simulink model "QAM"  (R2022b)
settings: Solver=VariableStepAuto  StartTime=0.0  StopTime=stop_time  RelTol=1e-3
libraries: commdigbbndam3 x2, commchan3 x1, commsink2 x1, commrandsrc3 x1
settings Model: Creator=g  LastModifiedBy=g

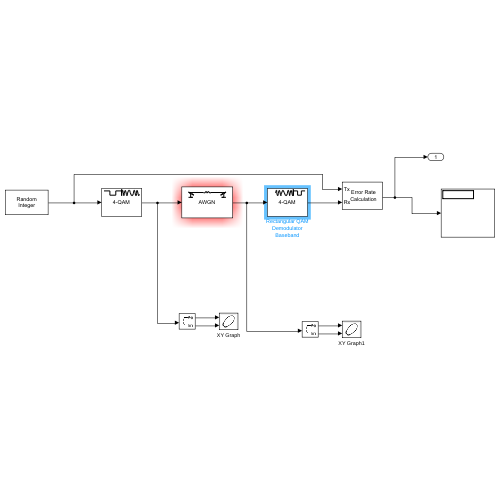
[thumbnail: Simulink's stored preview of the top-level diagram]
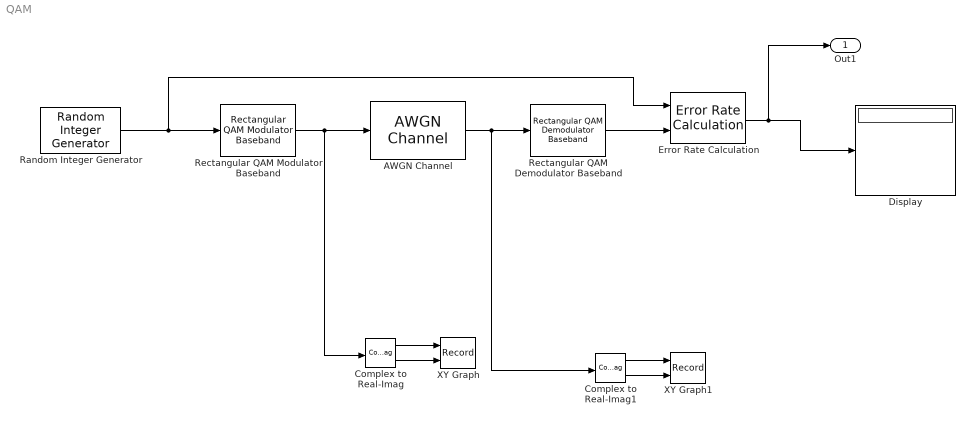
== system QAM ==
  AWGN Channel : commchan3/AWGN Channel  InputProcessing=Columns as channels (frame based)  seed=67  noiseMode="Signal to noise ratio  (Eb/No)"  EbNodB=Eb_No_db  EsNodB=10  SNRdB=10  bitsPerSym=2  Ps=1  Tsym=0.2  variance=1
  Complex to Real-Imag : ComplexToRealImag
  Complex to Real-Imag1 : ComplexToRealImag
  Display : Display
  Error Rate Calculation : commsink2/Error Rate Calculation  N=0  st_delay=0  cp_mode=Entire frame  subframe=[]  PMode=Port  WsName=ErrorVec  RsMode2=off  stop=off  numErr=100  maxBits=1e6
  Random Integer Generator : commrandsrc3/Random Integer Generator  SetSize=m_ary  SeedSource=Auto  Seed=0  SampleTime=0.1  SamplesPerFrame=1  OutputDataType=double  SimulateUsing=Interpreted execution
  Rectangular QAM Demodulator Baseband : commdigbbndam3/Rectangular QAM Demodulator Baseband  M=m_ary  OutType=Integer  DecType=Hard decision  VarSource=Dialog  Variance=1  Dec=Gray  Mapping=[0:15]  PowType=Average Power  MinDist=2  AvgPow=1  PeakPow=1  Ph=0  outDtype1=Inherit via internal rule  outDtype2=Inherit via internal rule  derotateFactorWordLen=16  derotateFactorDataTypeStr=Inherit: Same word length as input  derotateFactorLastDataTypeStr=Inherit: Same word length as input  denormFactorWordLen=16  denormFactorDataTypeStr=Inherit: Same word length as input  denormFactorLastDataTypeStr=Inherit: Same word length as input  prodOutWordLen=32  prodOutOverflowMode=Wrap  prodOutRoundingMode=Floor  prodOutOvFlMode=off  prodOutOvFlModeLastStrValue=off  sumWordLen=32
  Rectangular QAM Modulator Baseband : commdigbbndam3/Rectangular QAM Modulator Baseband  M=m_ary  InType=Integer  Enc=Gray  Mapping=[0:15]  PowType=Average Power  MinDist=2  AvgPow=1  PeakPow=1  Ph=0  outDtype=double  outWordLen=16  outUDDataType=sfix(16)  outFracLenMode=Best precision  outFracLen=15  outDataTypeStr=double  outLastDataTypeStr=double
  XY Graph : Record  FileSettingsInternal="{\"entries\":[{\"content\":{\"excelSettings\":{\"content\":{},\"type\":\"Streamout.ExcelSettings\"}},\"type\":\"Streamout.FileSettingStorage\",\"uuid\":\"e93c98fa-26f5-4796-a8ec-bd8ee0fda1c9\"}],\"packageUris\":[\"http://schema.mathworks.com/mf0/streamout_blocks/R2020a\"],\"version\":\"1.0\"}"  Layout=[1 1]  SignalsInternal="{\"entries\":[{\"content\":{\"signals\":[{\"content\":{\"blockPath\":[\"QAM/XY Graph\"],\"channel\":[],\"dimensions\":[1,1],\"domain\":\"QAM/XY Graph\",\"lineColor\":\"#a2142f\",\"plots\":[1],\"port\":1,\"sid\":[],\"signalID\":100,\"signalName\":\"Complex to\\nReal-Imag:1\"},\"type\":\"RecordBlkView.Signal\",\"uuid\":\"3696c84a-bfcc-42ec-836c-3c1d2b3aa4ae\"},{\"content\":{\"blockPath\":[\"QAM/XY Graph\"],\"channel\":[],\"dimensions\":[1,1],\"domain\":\"QAM/XY Graph\",\"lineColor\":\"#139fff\",\"plots\":[1],\"port\":2,\"sid\":[],\"signalID\":103,\"signalName\":\"Complex to\\nReal-Imag:2\"},\"type\":\"RecordBlkView.Signal\",\"uuid\":\"59295ec4-1a42-4058-9d3d-41e943421700\"}]},\"type\":\"RecordBlkView.InputSignals\",\"uuid\":\"316a87c3-4eb9-4bcf-83c6-6cfffa126bcd\"}],\"packageUris\":[\"http://schema.mathworks.com/mf0/streamout_blocks/R2020a\"],\"version\":\"1.0\"}"  VisualizationBindings="{\"xyplotplugin\":{\"info\":[{\"series\":[{\"bindingParametersList\":[{\"parameter\":\"X-Axis\",\"signalID\":100,\"signalName\":\"Complex to\\nReal-Imag:1\"},{\"parameter\":\"Y-Axis\",\"signalID\":103,\"signalName\":\"Complex to\\nReal-Imag:2\"}],\"seriesID\":36458}],\"subplotID\":1}]}}"  CompatibilityTag=XY
  XY Graph1 : Record  FileSettingsInternal="{\"entries\":[{\"content\":{\"excelSettings\":{\"content\":{},\"type\":\"Streamout.ExcelSettings\"}},\"type\":\"Streamout.FileSettingStorage\",\"uuid\":\"0223a079-f81d-4abb-aeb4-10d8bcb112ae\"}],\"packageUris\":[\"http://schema.mathworks.com/mf0/streamout_blocks/R2020a\"],\"version\":\"1.0\"}"  Layout=[1 1]  SignalsInternal="{\"entries\":[{\"content\":{\"signals\":[{\"content\":{\"blockPath\":[\"QAM/XY Graph1\"],\"channel\":[],\"dimensions\":[1,1],\"domain\":\"QAM/XY Graph1\",\"lineColor\":\"#a2142f\",\"plots\":[1],\"port\":1,\"sid\":[],\"signalID\":92,\"signalName\":\"Complex to\\nReal-Imag1:1\"},\"type\":\"RecordBlkView.Signal\",\"uuid\":\"dae8d86f-60ac-4c44-8e31-9bb592083225\"},{\"content\":{\"blockPath\":[\"QAM/XY Graph1\"],\"channel\":[],\"dimensions\":[1,1],\"domain\":\"QAM/XY Graph1\",\"lineColor\":\"#139fff\",\"plots\":[1],\"port\":2,\"sid\":[],\"signalID\":95,\"signalName\":\"Complex to\\nReal-Imag1:2\"},\"type\":\"RecordBlkView.Signal\",\"uuid\":\"623fe431-37a5-4f12-a841-dbf7a4b993fe\"}]},\"type\":\"RecordBlkView.InputSignals\",\"uuid\":\"b60af5d1-0e3b-4b2e-8d12-89979b68d21d\"}],\"packageUris\":[\"http://schema.mathworks.com/mf0/streamout_blocks/R2020a\"],\"version\":\"1.0\"}"  VisualizationBindings="{\"xyplotplugin\":{\"info\":[{\"series\":[{\"bindingParametersList\":[{\"parameter\":\"X-Axis\",\"signalID\":92,\"signalName\":\"Complex to\\nReal-Imag1:1\"},{\"parameter\":\"Y-Axis\",\"signalID\":95,\"signalName\":\"Complex to\\nReal-Imag1:2\"}],\"seriesID\":32705}],\"subplotID\":1}]}}"  CompatibilityTag=XY
  Out1 : Outport
  wires:
  Random Integer Generator/1 -> Rectangular QAM Modulator Baseband/1, Error Rate Calculation/1
  Rectangular QAM Modulator Baseband/1 -> Complex to Real-Imag/1, AWGN Channel/1
  AWGN Channel/1 -> Rectangular QAM Demodulator Baseband/1, Complex to Real-Imag1/1
  Rectangular QAM Demodulator Baseband/1 -> Error Rate Calculation/2
  Error Rate Calculation/1 -> Out1/1, Display/1
  Complex to Real-Imag/1 -> XY Graph/1
  Complex to Real-Imag/2 -> XY Graph/2
  Complex to Real-Imag1/1 -> XY Graph1/1
  Complex to Real-Imag1/2 -> XY Graph1/2
